simulink model "Michaels_CVModel_fast8"  (R2020a)
settings: Solver=ode23  StartTime=0.0  StopTime=30  RelTol=1e-2  EnableMultiTasking=on
model workspace (MAT data in the model file):
  Eao = 1.88
  Eesla = 0.58
  Eeslvf = 5.2
  Eesra = 0.63
  Eesrvf = 1.75
  Emaxspt = 48.75
  Epa = 0.15
  Epu = 0.04
  Esa = 0.37
  Esv = 0.013
  Evc = 0.03
  GpLV = 0
  GpRR = 11
  GpRV = 0
  GpRsa = 0
  GpV0 = 0
  GsLV = 0.007
  GsRR = 11
  GsRV = 0.022
  GsRsa = -0.05
  GsV0 = 31
  Ka = 4.4
  Lao = 0.0022
  Lav = 0.000354
  Lmt = 7.697e-05
  Lpa = 7.697e-05
  Lpv = 0.0001043
  Ltc = 8.009e-05
  P0la = 0.5
  P0lvf = 0.98
  P0pcd = 0.5
  P0ra = 0.5
  P0rvf = 0.91
  P0spt = 0.46
  PV : AO (value not decoded)
  PVao = [327.9; 100.9]
  Rao = 0.28
  Rav = 0.02
  Rla2pu = 0.5
  Rmt = 0.01
  Rpa = 0.12
  Rpa_Vals = 0.12
  Rpu = 0.006
  Rpv = 0.02
  Rra = 0.012
  Rsa = 0.74
  Rsv = 0.12
  Rtc = 0.01
  Tc = 1
  Tsys0 = 0.6
  V0la = 30
  V0lvf = 45
  V0pcd = 200
  V0ra = 25
  V0rvf = 50
  V0spt = 10
  Vdla = 15
  Vdlvf = 16
  Vdra = 15
  Vdrvf = 40
  Vdspt = 10
  Vlv0 = 100
  Vperi = 51
  Vrv0 = 105
  Vuao = 260.8
  Vupa = 91
  Vupu = 132
  Vusa = 287.4
  Vusv = 1976.1
  Vuvc = 136.17
  amin = -2
  artBrLVcontConti = []
  artBrLVcontDigi = [0 0 0 0 0 0 0 0 0 0 0 0 ... (240 elements, 1x240)]
  artBrRRConti = []
  artBrRRDigi = [0 0 0 0 0 0 0 0 0 0 1.57142857143 3.14285714286 ... (240 elements, 1x240)]
  artBrRVcontConti = []
  artBrRVcontDigi = [0 0 0 0 0 0 0 0 0 0 0 0 ... (240 elements, 1x240)]
  artBrRsaConti = []
  artBrRsaDigi = [0 0 0 0 0 0 0 0 0 0 0 0 ... (480 elements, 1x480)]
  artBrV0Conti = []
  artBrV0Digi = [0 0 0 0 0 0 0 0 0 0 0 0 ... (640 elements, 1x640)]
  atriumA = 1
  baroSampFreq = 16
  cP0la = 0.5
  cP0lvf = 0.98
  cP0ra = 0.5
  cP0rvf = 0.91
  cT = 1
  cVtotal = 5400
  clambdala = 0.13
  clambdalvf = 0.028
  clambdara = 0.13
  clambdarvf = 0.028
  deac = 0.0004
  ksys = 0.075
  lambdala = 0.065
  lambdalvf = 0.042
  lambdapcd = 0.005
  lambdara = 0.065
  lambdarvf = 0.028
  lambdaspt = 0.4
  pThor = 0
  params : object (value not decoded)
  sampleTime = 0.005
  svcPressureChange_MCS = 0
  svrMult = 1
  tStepOn = 1000000000
  t_baroOn = 1000000
  t_testBed_start = 1000000
  venk1 = 0.5
  venk2 = 0.5
symbols that are objects in the model workspace (value not decoded): PV
undefined symbols (not defined in the file): dfilt
libraries: simulink x85, fl_lib x39, nesl_utility x24, cstblocks x9, dspstat3 x9, dspobslib x5, SimscapeFluids_lib x5, sh_lib x1
(part 2 of 5)

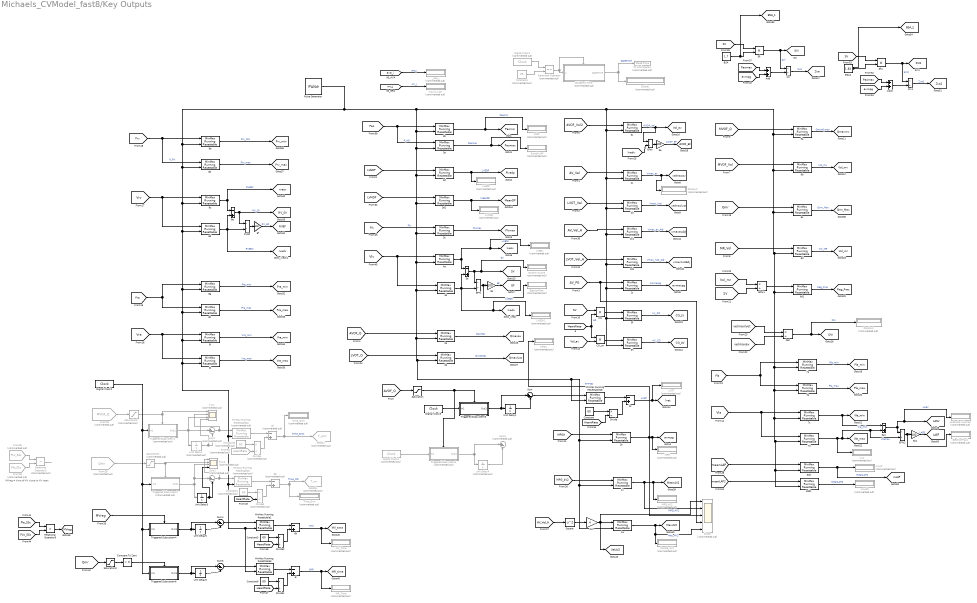
== system Michaels_CVModel_fast8/Key Outputs ==
  note: MRreg = time of MV close to MV open
  00 Date & Time : Subsystem  Commented=on
  1a : Sum  Description=1a  Inputs=-+
  1b : simulink/Math Operations/MinMax Running Resettable  Description=1b  Function=max  vinit=0
  1c : simulink/Math Operations/MinMax Running Resettable  Description=1c  Function=max  vinit=0
  1v : simulink/Math Operations/MinMax Running Resettable  Description=1b  Function=max  vinit=0
  1w : simulink/Math Operations/MinMax Running Resettable  Description=1b  Function=max  vinit=0
  1zv : Product  Inputs=*/
  1zv1 : Product  Inputs=*/
  2a : simulink/Math Operations/MinMax Running Resettable  Description=2a  Function=max  vinit=0
  2b : simulink/Math Operations/MinMax Running Resettable  Description=2b  Function=max  vinit=0
  2c : simulink/Math Operations/MinMax Running Resettable  Description=2c  Function=max  vinit=0
  2c1 : simulink/Math Operations/MinMax Running Resettable  Description=2c  Function=max  vinit=0
  2d : simulink/Math Operations/MinMax Running Resettable  Description=2d  Function=max  vinit=0
  2d1 : simulink/Math Operations/MinMax Running Resettable  Description=2d  Function=max  vinit=0
  2e0 : Product  Description=2e  Inputs=*/
  3a : simulink/Math Operations/MinMax Running Resettable  Description=3a  Function=max  vinit=0
  3b : simulink/Math Operations/MinMax Running Resettable  Description=3b  Function=min  vinit=250
  3c : simulink/Math Operations/MinMax Running Resettable  Description=3c  Function=max  vinit=0
  3d : simulink/Math Operations/MinMax Running Resettable  Description=3d  Function=max  vinit=0
  3d1 : simulink/Math Operations/MinMax Running Resettable  Description=3d  Function=max  vinit=0
  3dd : simulink/Math Operations/MinMax Running Resettable  Description=7d  Function=max  vinit=0
  3dd1 : simulink/Math Operations/MinMax Running Resettable  Description=7d  Function=max  vinit=0
  4V2 : Gain  Gain=4
  4a : simulink/Math Operations/MinMax Running Resettable  Description=4a  Function=min  vinit=250
  4b : simulink/Math Operations/MinMax Running Resettable  Description=4b  Function=max  vinit=0
  5a : Sum  Description=5a  Inputs=-+
  5a1 : Sum  Description=5a  Inputs=-+
  5b : Gain  Description=5b  Gain=100
  5b1 : Gain  Description=5b  Gain=100
  5c : simulink/Math Operations/MinMax Running Resettable  Description=5c  Function=max  vinit=0
  5e : Gain  Description=5e  Gain=100
  5f : simulink/Math Operations/MinMax Running Resettable  Description=5f  Function=max  vinit=0
  5fi : Product  Inputs=**
  5fi1 : Product  Inputs=**
  5h : simulink/Math Operations/MinMax Running Resettable  Description=5h  Function=max  vinit=0
  6a : simulink/Math Operations/MinMax Running Resettable  Description=6a  Function=max  vinit=0
  6b : simulink/Math Operations/MinMax Running Resettable  Description=6b  Function=max  vinit=0
  6c : simulink/Math Operations/MinMax Running Resettable  Description=6a  Function=max  vinit=0
  6d : simulink/Math Operations/MinMax Running Resettable  Description=6c  Function=max  vinit=0
  6d1 : simulink/Math Operations/MinMax Running Resettable  Description=6d  Function=max  vinit=0
  6f : Sum  Description=6f  Commented=on  Inputs=-+
  6g : Sum  Description=6g  Commented=on  Inputs=-+
  6h : Sum  Description=1a  Inputs=-+
  6i : Sum  Description=1a  Inputs=-+
  7a : simulink/Math Operations/MinMax Running Resettable  Description=7a  Function=min  vinit=250
  7b : simulink/Math Operations/MinMax Running Resettable  Description=7b  Function=max  vinit=0
  7c : simulink/Math Operations/MinMax Running Resettable  Description=7c  Function=min  vinit=250
  7d : simulink/Math Operations/MinMax Running Resettable  Description=7d  Function=max  vinit=0
  8a : simulink/Math Operations/MinMax Running Resettable  Description=3b  Function=min  vinit=250
  8b : simulink/Math Operations/MinMax Running Resettable  Description=3a  Function=max  vinit=0
  8c : simulink/Math Operations/MinMax Running Resettable  Description=4a  Function=min  vinit=250
  8d : simulink/Math Operations/MinMax Running Resettable  Description=4b  Function=max  vinit=0
  8e : Sum  Description=5a  Inputs=-+
  8f : Gain  Description=5b  Gain=100
  8g : simulink/Math Operations/MinMax Running Resettable  Description=7a  Function=min  vinit=250
  8h : simulink/Math Operations/MinMax Running Resettable  Description=7b  Function=max  vinit=0
  8i : simulink/Math Operations/MinMax Running Resettable  Description=7c  Function=min  vinit=250
  8j : simulink/Math Operations/MinMax Running Resettable  Description=7d  Function=max  vinit=0
  Add : Sum
  Add1 : Sum
  BSA : Constant  Value=1.7  SampleTime=0.001
  BSA2 : Constant  Value=1.83  SampleTime=0.001
  CO : Product  Inputs=**
  CO_av : Product  Inputs=**
  Compare To Zero : simulink/Logic and Bit Operations/Compare To Zero  relop=>  OutDataTypeStr=boolean  ZeroCross=off
  Constant : Constant  Value=60  SampleTime=0.001
  Constant1 : Constant  Commented=on  Value=60  SampleTime=0.001
  Constant3 : Constant  Value=60  SampleTime=0.001
  Constant4 : Constant  Commented=on  Value=25  SampleTime=0.001
  Constant5 : Constant  Commented=on  Value=60  SampleTime=0.001
  Constant6 : Constant  Value=60  SampleTime=0.001
  D BP : Display  Commented=on
  Digital Clock1 : DigitalClock  Commented=on  SampleTime=0.001
  Digital Clock2 : DigitalClock  SampleTime=0.001
  Digital Clock3 : DigitalClock  SampleTime=0.001
  Digital Clock4 : DigitalClock  Commented=on  SampleTime=0.001
  Display : Display  Commented=on
  Display1 : Display  Commented=on
  Display2 : Display  Commented=on
  Divide : Product  Inputs=*/
  Divide1 : Product  Inputs=*/
  Divide2 : Product  Inputs=*/
  Divide3 : Product  Commented=on  Inputs=*/
  Divide4 : Product  Commented=on  Inputs=*/
  EF% : Product  Inputs=*/
  EF%1 : Product  Inputs=*/
  EF%2 : Product  Inputs=*/
  EFav : Product  Inputs=*/
  EjectionFrac : Display  Commented=on
  EjectionFrac1 : Display  Commented=on
  From28 : From  Commented=on  GotoTag=Qmr  TagVisibility=global
  From29 : From  Commented=on  GotoTag=MVOF_Q  TagVisibility=global
  From35 : From  Commented=on  GotoTag=PLV_SSc  TagVisibility=global
  From36 : From  Commented=on  GotoTag=Pla_SSc  TagVisibility=global
      settings: CloseFcn=tagdialog Close
  From50 : From  Commented=on  GotoTag=HeartRate  TagVisibility=global
  Goto15 : Goto  Commented=on  GotoTag=T_mr  TagVisibility=global
  Goto17 : Goto  Commented=on  GotoTag=T_qmt  TagVisibility=global
  LAStroke Volume1 : Display  Commented=on
  LVEDP : Display  Commented=on
  LVEDV1 : Display  Commented=on
  LVESV : Display  Commented=on
  LVET : Display  Commented=on
  LVMDP : Display  Commented=on
  MPG : Display  Commented=on
  MPG1 : Display  Commented=on
  MPG_4V2 : Display  Commented=on
  MR_Time : Display  Commented=on
  MV_Time : Display  Commented=on
  MaxPG_4V2 : Display  Commented=on
  MinMax Running Resettable1 : simulink/Math Operations/MinMax Running Resettable  Function=max  vinit=0
  MinMax Running Resettable18 : simulink/Math Operations/MinMax Running Resettable  Function=max  vinit=0
  MinMax Running Resettable2 : simulink/Math Operations/MinMax Running Resettable  Commented=on  Function=max  vinit=0
  MinMax Running Resettable22 : simulink/Math Operations/MinMax Running Resettable  Commented=on  Function=max  vinit=0
  MinMax Running Resettable3 : simulink/Math Operations/MinMax Running Resettable  Function=max  vinit=0
  Pulse Generator : DiscretePulseGenerator  PulseType=Time based  Period=20  PhaseDelay=28.7
  RVEF : Product  Inputs=*/
  Relational Operator : RelationalOperator  Commented=on  Operator===  OutDataTypeStr=boolean  RndMeth=Simplest
  Relational Operator3 : RelationalOperator  Commented=on  Operator=>  OutDataTypeStr=boolean  RndMeth=Simplest
  Relational Operator5 : RelationalOperator  Operator=>  OutDataTypeStr=boolean  ZeroCross=off  RndMeth=Simplest
  Saturation : Saturate  UpperLimit=inf  LowerLimit=0  RndMeth=Ceiling
  Saturation1 : Saturate  Commented=on  UpperLimit=inf  LowerLimit=0  RndMeth=Ceiling
  Saturation2 : Saturate  UpperLimit=inf  LowerLimit=0  RndMeth=Ceiling
  Saturation3 : Saturate  Commented=on  UpperLimit=inf  LowerLimit=0  RndMeth=Ceiling
  Scope : Scope  Commented=on  NumInputPorts=5
  Square : Math  Operator=square  SaturateOnIntegerOverflow=on
  Stroke Volume : Display  Commented=on
  Sum : Sum  Inputs=|+-
  Sum1 : Sum  Commented=on  Inputs=|+-
  Sum2 : Sum  Commented=on  Inputs=|+-
  Sum3 : Sum  Commented=on  Inputs=|+-
  Sum4 : Sum  Inputs=|+-
  Sum5 : Sum  Inputs=|+-
  Systolic BP : Display  Commented=on
  T MV : Scope  Commented=on  NumInputPorts=4
  Time_Qmr : Display  Commented=on
  Time_Qmt : Display  Commented=on
  Tmr0 : Scope  Commented=on  NumInputPorts=4
  To Workspace1 : ToWorkspace  Commented=on  VariableName=DateTime  SaveFormat=Structure  SampleTime=1
      settings: MaxDataPoints=1  Save2DSignal=2-D array (concatenate along first dimension)
  Triggered Subsystem1 : Subsystem  Commented=on  TreatAsAtomicUnit=on
  Triggered Subsystem2 : Subsystem  Commented=on  TreatAsAtomicUnit=on
  Triggered Subsystem3 : Subsystem  Commented=on  TreatAsAtomicUnit=on
  Triggered Subsystem4 : Subsystem  TreatAsAtomicUnit=on
  Triggered Subsystem5 : Subsystem  TreatAsAtomicUnit=on
  Triggered Subsystem6 : Subsystem  TreatAsAtomicUnit=on
  Unit Delay{1,3,5..6} (4 alike) : UnitDelay  SampleTime=0.001
  Unit Delay2 : UnitDelay  Commented=on  SampleTime=0.001
  Unit Delay4 : UnitDelay  Commented=on  SampleTime=-1
  VLA : Display  Commented=on
  _ava_i : Display  Commented=on
  mLAP : Display  Commented=on
  mLAP2 : Display  Commented=on
  max(u,y)20 : Display  Commented=on
  tag scope: AVOF_EF=global, BSA_1=global, BSA_2=global, CO_AV=global, CO_LV=global, DVI=global, EF=global, LAEF=global, LASV=global, MR_time=global, MV_time=global, MVreg=global, Max4V2=global, Mean4V2=global, MeanDP=global, Paomax=global, Paomin=global, Pla_max=global, Pla_min=global, Plvedp=global, Plvmax=global, Pra_max=global, Pra_min=global, Prv_max=global, Prv_min=global, Qmaxav=global, Qmaxlvot=global, Qmaxmv=global, Qmr_Max=global, RVEF=global, RV_SV=global, Reg_Frac=global, SV=global, SVI2=global, SVI=global, Vel4V2=global, Vla_max=global, Vla_min=global, Vol_av=global, Vol_mr=global, Vol_mv=global, Vra_max=global, Vra_min=global, Zva2=global, Zva=global, avmaxpg=global, avmpg=global, lvedv=global, lvesv=global, lvet=global, mLAP=global, rvedv=global, rvesv=global, velmaxav=global, velmaxlvot=global, vmaxavAdj=global, vmaxlvotAdj=global
  wires:
  3c/1 -> [Plvmax]  "Plvmax"
  [Vlv] -> 4a/1, 4b/1
  4a/1 -> 5a/1, LVESV/1, [lvesv]  "LVESV"
  [LVOT_Vel] -> 2d/1
  [AV_Vel] -> 2c/1
  2a/1 -> [Qmaxav]  "QavMax"
  [AV_PG] -> Scope/4, 1c/1
  3a/1 -> Systolic BP/1, [Paomax]  "Paomax"
  2c/1 -> Display2/1, [velmaxav]  "Vmax_av"
  4b/1 -> 5a/2, LVEDV1/1, [lvedv], EF%/2  "LVEDV"
  [Plv] -> 3c/1  "Plv"
  3b/1 -> D BP/1, [Paomin]  "Paomin"
  [Pao] -> 3a/1, 3b/1  "P_AO"
  1c/1 -> [avmaxpg]  "AVmaxpg"
  6b/1 -> [Vol_mv]  "Vol_mv"
  6d/1 -> [Vol_mr]  "Vol_MR"
  5c/1 -> EFav/1, [Vol_av]  "AVOF_vol"
  [MVOF_Vol] -> 6b/1
  [AVOF_Vol2] -> 5c/1
  6a/1 -> [Qmaxmv]  "Qmvof_max"
  Triggered Subsystem5/1(Out1) -> Sum/1, Unit Delay1/1
  Unit Delay1/1 -> Sum/2
  [Pla] -> 7a/1, 7b/1
  7a/1 -> [Pla_min]  "Pla_min"
  7b/1 -> [Pla_max]  "Pla_max"
  [Vla] -> 7d/1, 7c/1
  Sum1/1 -> T MV/2, MinMax Running Resettable22/1
  Unit Delay2/1 -> T MV/4, Sum1/2
  [MVOF_Q] -> 6a/1
  Triggered Subsystem1/1(Out1) -> Unit Delay2/1, T MV/3, Sum1/1
  Triggered Subsystem2/1(Out1) -> Unit Delay3/1, Tmr0/3, Sum2/1
  [MR_Vol] -> 6d/1
  Unit Delay3/1 -> Tmr0/4, Sum2/2
  Sum2/1 -> MinMax Running Resettable2/1, Tmr0/1
  [AVOF_Q] -> Saturation/1
  MinMax Running Resettable18/1 -> 1a/1
  Sum/1 -> MinMax Running Resettable18/1
  [LVEDP] -> 3d/1
  3d/1 -> LVEDP/1, [Plvedp]  "LVEDP"
  Digital Clock4/1 -> Triggered Subsystem3/1(In1)
  Unit Delay4/1 -> Sum3/2
  Triggered Subsystem3/1(Out1) -> Sum3/1, Unit Delay4/1
  Constant/1 -> Divide/1
  1a/1 -> LVET/1, [lvet]  "LVET"
  [MPGX] -> 1b/1
  1b/1 -> MPG1/1, Scope/3, MPG/1, [avmpg]  "avmpg"
  2d/1 -> [velmaxlvot]  "Vmax_lvot"
  MinMax Running Resettable2/1 -> 6g/1
  Saturation1/1 -> Tmr0/2, Triggered Subsystem2/Trigger
  MinMax Running Resettable22/1 -> 6f/1
  Digital Clock3/1 -> Triggered Subsystem5/1(In1)
  5b/1 -> [EF]  "EF"
  EF%/1 -> EjectionFrac/1, 5b/1
  5a/1 -> EF%/1, [SV], Stroke Volume/1  "SV"
  [mr_j] -> max(u,y)20/1  "mr_j"
  [ava_i] -> _ava_i/1  "ava_i"
  6g/1 -> Goto15/1, Time_Qmr/1  "Time_MR"
  6f/1 -> Time_Qmt/1, Goto17/1  "Time_Qmt"
  7c/1 -> 5a1/1, [Vla_min]  "Vla_min"
  [AVOF_Q] -> 2a/1
  5f/1 -> [CO_LV]  "LV_CO"
  [SV] -> CO/1
  [Vol_av] -> CO_av/2
  5h/1 -> [CO_AV]  "AV_CO"
  [HeartRate] -> CO/2, CO_av/1  "HR"
  CO_av/1 -> 5h/1
  CO/1 -> 5f/1
  6d1/1 -> [Reg_Frac]  "Reg_Frac"
  EF%1/1 -> 6d1/1
  [Vol_mr] -> EF%1/1
  [SV] -> EF%1/2
  [velmaxlvot] -> 2e0/1
  [velmaxav] -> 2e0/2
  2e0/1 -> Display1/1, [DVI]  "DVI"
  [LVOT_Q] -> 2b/1
  2b/1 -> [Qmaxlvot]  "QlvotMax"
  5e/1 -> [AVOF_EF]  "AVOF_EF"
  EFav/1 -> 5e/1
  [lvedv] -> EFav/2
  8e/1 -> RVEF/1, [RV_SV]  "RV_SV"
  RVEF/1 -> 8f/1
  8d/1 -> 8e/2, [rvedv], RVEF/2  "RVEDV"
  8c/1 -> 8e/1, [rvesv]  "RVESV"
  8f/1 -> [RVEF]  "RV_EF"
  [Vrv] -> 8c/1, 8d/1
  8h/1 -> [Pra_max]  "Pra_max"
  [Pra] -> 8g/1, 8h/1
  8g/1 -> [Pra_min]  "Pra_min"
  [Vra] -> 8j/1, 8i/1
  8i/1 -> [Vra_min]  "Vra_min"
  8j/1 -> [Vra_max]  "Vra_max"
  [Prv] -> 8a/1, 8b/1  "P_RV"
  8a/1 -> [Prv_min]  "Prv_Min"
  8b/1 -> [Prv_max]  "Prv_max"
  From29/1 -> Saturation3/1
  From28/1 -> Saturation1/1
  [Qmr] -> 6c/1
  6c/1 -> [Qmr_Max]  "Qmr_Max"
  1v/1 -> Scope/2, [Mean4V2], MPG_4V2/1  "MPG_4V2"
  [MPG_4V2] -> 1v/1
  [AV_Vel_A] -> Square/1
  1w/1 -> Scope/5, MaxPG_4V2/1, [Max4V2]  "Max_4V2"
  4V2/1 -> [Vel4V2], Scope/1, 1w/1
  Square/1 -> 4V2/1
  2d1/1 -> [vmaxlvotAdj]  "Vmax_lvot_Adj"
  2c1/1 -> [vmaxavAdj]  "Vmax_av_Adj"
  [AV_Vel_A] -> 2c1/1
  [LVOT_Vel_A] -> 2d1/1
  3d1/1 -> [MeanDP], LVMDP/1  "meanDP"
  [LVMDP] -> 3d1/1
  Digital Clock1/1 -> Relational Operator/1
  Relational Operator/1 -> 00 Date & Time/Enable, 00 Date & Time/1(u)
  Constant4/1 -> Relational Operator/2
  00 Date & Time/1(DateTime) -> To Workspace1/1, Display/1  "DateTime"
  From35/1 -> Relational Operator3/1
  From36/1 -> Relational Operator3/2
  Relational Operator3/1 -> ?
  Saturation3/1 -> Triggered Subsystem1/Trigger, T MV/1
  6h/1 -> [MV_time], MV_Time/1  "tMV"
  [MVreg] -> Triggered Subsystem4/Enable
  Sum4/1 -> MinMax Running Resettable1/1
  MinMax Running Resettable1/1 -> 6h/1
  Unit Delay5/1 -> Sum4/2
  Triggered Subsystem4/1(Out1) -> Unit Delay5/1, Sum4/1
  [PLV_SSc] -> Relational Operator5/2
  [Pla_SSc] -> Relational Operator5/1
  Relational Operator5/1 -> [MVreg]
  Triggered Subsystem6/1(Out1) -> Sum5/1, Unit Delay6/1
  Unit Delay6/1 -> Sum5/2
  MinMax Running Resettable3/1 -> 6i/1
  Sum5/1 -> MinMax Running Resettable3/1
  Compare To Zero/1 -> Triggered Subsystem6/Enable
  6i/1 -> MR_Time/1, [MR_time]  "tMR"
  Digital Clock2/1 -> Triggered Subsystem6/1(In1), Triggered Subsystem4/1(In1), Triggered Subsystem2/1(In1), Triggered Subsystem1/1(In1)
  5fi/1 -> 1zv/1, [SVI]  "SVI"
  Add/1 -> 1zv/2
  BSA/1 -> [BSA_1], 5fi/2
  [SV] -> 5fi/1
  1zv/1 -> [Zva]  "Zva"
  [Paomax] -> Add/1
  [avmpg] -> Add/2
  [Qmr] -> Saturation2/1
  Saturation2/1 -> Compare To Zero/1
  Saturation/1 -> Triggered Subsystem5/Enable, Triggered Subsystem3/Trigger
  [HeartRate] -> Divide/2
  Divide/1 -> 1a/2
  5b1/1 -> [LAEF]  "LAEF"
  5a1/1 -> [LASV], LAStroke Volume1/1, EF%2/1  "LASV"
  7d/1 -> VLA/1, [Vla_max], EF%2/2, 5a1/2  "Vlamax"
  EF%2/1 -> EjectionFrac1/1, 5b1/1
  [meanLAP] -> 3dd/1
  3dd/1 -> [mLAP], mLAP/1  "meanLAP1"
  Divide1/1 -> 6i/2
  Constant6/1 -> Divide1/1
  [HeartRate] -> Divide1/2
  [HeartRate] -> Divide2/2
  Constant3/1 -> Divide2/1
  Divide2/1 -> 6h/2
  Divide3/1 -> 6g/2
  Constant1/1 -> Divide3/1
  [HeartRate] -> Divide3/2
  From50/1 -> Divide4/2
  Constant5/1 -> Divide4/1
  Divide4/1 -> 6f/2
  3dd1/1 -> mLAP2/1  "meanLAP2"
  [meanLAP2] -> 3dd1/1
  Pulse Generator/1 -> 3d1/2, 4a/2, 4b/2, 2a/2, MinMax Running Resettable18/2, 1v/2, 1w/2, 1b/2, 2b/2, 3c/2, 3d/2, 3a/2, 3b/2, 6c/2, 6d/2, 6d1/2, 7a/2, 7b/2, 3dd1/2, 3dd/2, 7d/2, 7c/2, 6b/2, 6a/2, 5c/2, 2d/2, 2c1/2, 2d1/2, 1c/2, 5h/2, 5f/2, 2c/2, 8g/2, 8h/2, MinMax Running Resettable22/2, MinMax Running Resettable1/2, MinMax Running Resettable3/2, MinMax Running Resettable2/2, 8j/2, 8i/2, 8d/2, 8c/2, 8b/2, 8a/2
  [avmpg] -> Add1/2
  [Paomax] -> Add1/1
  1zv1/1 -> [Zva2]  "Zva2"
  [SV] -> 5fi1/1
  Add1/1 -> 1zv1/2
  5fi1/1 -> [SVI2], 1zv1/1  "SVI2"
  BSA2/1 -> [BSA_2], 5fi1/2

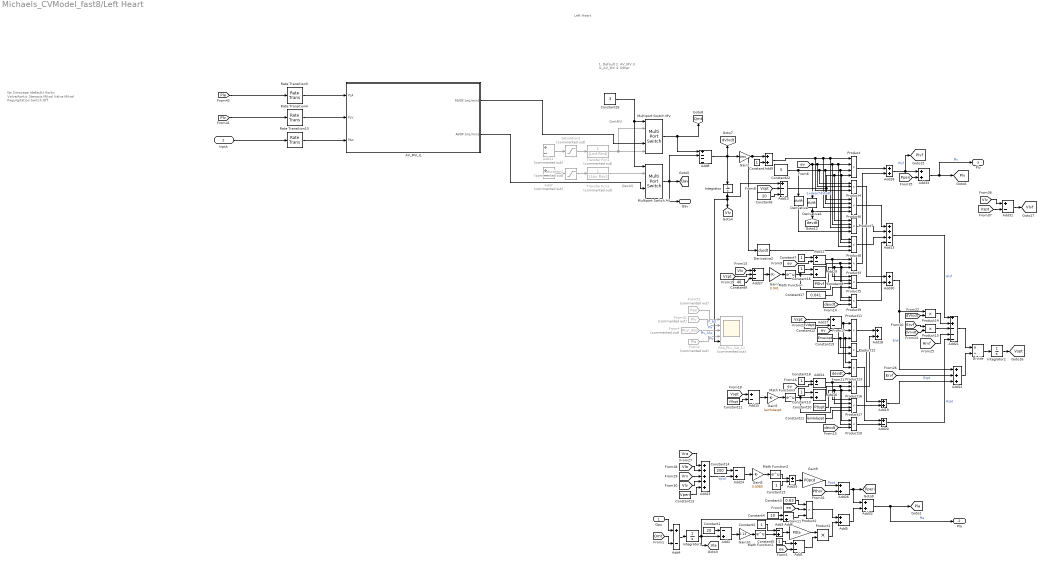
== system Michaels_CVModel_fast8/Left Heart ==
  note: No Simscape (default)
      | Aortic Valve/Aortic Stenosis
      | Mitral Valve
      | Mitral Regurgitation
      | Switch Off
  note: QavAS
  note: Left Heart
  note: QmtMV
  note: 1. Default
      | 2. AV_MV
      | 3. IL_AV_MV
      | 4. Other
  Qpu : Inport
  Input : Inport  Port=2
  AV_MV_IL : Subsystem
  Add{1,4,12,14..15,17,20,25,31} (9 alike) : Sum  Inputs=+-
  Add10 : Sum  Inputs=+--
  Add11 : Sum  Commented=on  Inputs=+-
  Add13 : Sum  Inputs=+++-
  Add{2..3,6,16,24,29} (6 alike) : Sum  Inputs=-+
  Add{5,9,18..19,26,28,30,32..33} (9 alike) : Sum
  Add21 : Sum  Inputs=++---
  Add22 : Sum  Inputs=+++
  Add23 : Sum  Inputs=+++++
  Add27 : Sum  Inputs=+--
  Add7 : Sum  Commented=on  Inputs=+-
  Add8 : Sum  Inputs=+---
  Constant{,2,5,7,10,15..16,18} (8 alike) : Constant
  Constant1 : Constant  Value=20
  Constant11 : Constant  Value=lambdaspt
  Constant12 : Constant  Value=Vdspt
  Constant13 : Constant  Value=Vperi
  Constant14 : Constant  Value=200
  Constant17 : Constant  Value=0.041
  Constant19 : Constant  Value=Emaxspt
  Constant20 : Constant  Value=P0spt
  Constant21 : Constant  Value=V0spt
  Constant22 : Constant  Value=5
  Constant26 : Constant  Value=3  SampleTime=-1
  Constant3 : Constant  Value=0.63
  Constant4 : Constant  Value=10
  Constant6 : Constant  Value=20
  Constant8 : Constant  Value=P0lvf
  Constant9 : Constant  Value=40
  Derivative : Derivative
  Derivative1 : Derivative
  Derivative2 : Derivative
  Divide : Product  Inputs=*/
  From2 : From  Commented=on  GotoTag=Pla  TagVisibility=global
      settings: CloseFcn=tagdialog Close
  From32 : From  Commented=on  GotoTag=Plv  TagVisibility=global
      settings: CloseFcn=tagdialog Close
  From4 : From  Commented=on  GotoTag=PLV_SSc  TagVisibility=global
      settings: CloseFcn=tagdialog Close
  From51 : From  Commented=on  GotoTag=Pao  TagVisibility=global
      settings: CloseFcn=tagdialog Close
  Gain10 : Gain  Gain=0.13
  Gain11 : Gain  Gain=P0la
  Gain2 : Gain  Gain=deac
  Gain3 : Gain  Gain=0.041
  Gain5 : Gain  Gain=lambdaspt
  Gain8 : Gain  Gain=0.0085
  Gain9 : Gain  Gain=P0pcd
  Integrator : Integrator  InitialCondition=140
  Integrator1 : Integrator  InitialCondition=40
  Integrator2 : Integrator  InitialCondition=20
  Math Function{,1..3} (4 alike) : Math  SignedPower=on  SaturateOnIntegerOverflow=on
  Multiport Switch AV : MultiPortSwitch  Inputs=4
  Multiport Switch MV : MultiPortSwitch  Inputs=4
  PAo_PLv_Vol_Lv : Scope  Commented=on  NumInputPorts=5
  Product{,5..8,17} (6 alike) : Product  Inputs=4  RndMeth=Zero
  Product{1,12,14..15} (4 alike) : Product  RndMeth=Zero
  Product{2..4,9..11,13,16} (8 alike) : Product  Inputs=3  RndMeth=Zero
  Rate Transition10 : RateTransition  OutPortSampleTimeMultiple=0.0  OutPortSampleTime=0.001
  Rate Transition3 : RateTransition  OutPortSampleTimeMultiple=0.0  OutPortSampleTime=0.001
  Rate Transition4 : RateTransition  OutPortSampleTimeMultiple=0.0  OutPortSampleTime=0.001
  Saturation1 : Saturate  Commented=on  UpperLimit=Inf  LowerLimit=0
  Saturation2 : Saturate  Commented=on  UpperLimit=Inf  LowerLimit=0
  Transfer Fcn1 : TransferFcn  Commented=on  Numerator=1  Denominator=[Lmt Rmt]
  Transfer Fcn2 : TransferFcn  Commented=on  Numerator=1  Denominator=[Lav Rav]
  Qav : Outport
  Pla : Outport  Port=2
  Plv : Outport  Port=3
  tag scope: Pla=global, Plv=global, Plvf=global, Pperi=global, Qav=global, Qmt=global, Vla=global, Vlv=global, Vlvf=global, Vspt=global, dVlvdt=global, devdt=global
  wires:
  Gain9/1 -> Add26/1  "Ppcd"
  [Pthor] -> Add26/2
  Add26/1 -> [Pperi], Add32/1
  Gain8/1 -> Math Function2/1
  Add24/1 -> Gain8/1
  Math Function2/1 -> Add25/1
  Constant15/1 -> Add25/2
  Add25/1 -> Gain9/1
  Math Function1/1 -> Add3/2
  Add3/1 -> Gain11/1
  Gain10/1 -> Math Function1/1
  Add2/1 -> Gain10/1
  Integrator1/1 -> Add2/2, Add6/2, [Vla]
  Constant1/1 -> Add2/1
  Add4/1 -> Integrator1/1
  Qpu/1 -> Add4/1
  [Qmt] -> Add4/2
  Constant2/1 -> Add3/1
  Constant4/1 -> Add6/1
  Add6/1 -> Product2/3
  [ea] -> Product2/2
  Constant3/1 -> Product2/1
  Product2/1 -> Add5/1
  Add5/1 -> Add32/2
  Add32/1 -> Pla/1, [Pla]  "Pla"
  Constant14/1 -> Add24/1
  [Vra] -> Add23/1
  [Vla] -> Add23/2
  [Vrv] -> Add23/3
  [Vlv] -> Add23/4
  Constant13/1 -> Add23/5
  Add23/1 -> Add24/2  "Vpcd"
  Gain11/1 -> Product1/1
  [ea] -> Add1/2
  Constant5/1 -> Add1/1
  Add1/1 -> Product1/2
  Product1/1 -> Add5/2
  Constant/1 -> Add9/2
  Gain2/1 -> Derivative2/1, Add9/1
  Add9/1 -> Product4/3, Product6/3, Product7/3, Product/1  "1+deac*dVlvdt"
  [ev] -> Product4/2, Product7/2, Product/2, Product8/3, Derivative1/1
  [Vspt] -> Add10/2
  Add10/1 -> Product7/1, Product/4, Product8/1, Product6/1
  Constant7/1 -> Add12/1
  Constant22/1 -> Product4/1, Product6/2, Product/3, Product8/2, Derivative/1
  [ev] -> Add12/2
  Product/1 -> Add28/1
  Product3/1 -> Add28/2
  Add28/1 -> Add33/1, [Plvf]  "Plvf"
  [Vlv] -> Add27/1
  [Vspt] -> Add27/2
  Constant9/1 -> Add27/3
  Gain3/1 -> Math Function/1
  Add27/1 -> Gain3/1
  Constant16/1 -> Add29/1
  Math Function/1 -> Add29/2, Product5/3
  Constant17/1 -> Product5/4
  Product4/1 -> Add30/1
  Product5/1 -> Add30/2
  Add30/1 -> Product14/1, Add22/1  "Elvf"
  Derivative1/1 -> Product6/4, [devdt]
  Derivative/1 -> Product7/4
  Constant8/1 -> Product5/2, Product3/3, Product9/1
  Add12/1 -> Product3/1, Product5/1
  Add29/1 -> Product3/2, Product9/2
  [devdt] -> Product9/3
  Product6/1 -> Add13/1
  Product7/1 -> Add13/2
  Product9/1 -> Add13/4
  Product8/1 -> Add13/3
  Add13/1 -> Add21/1  "Hlvf"
  Constant18/1 -> Add14/1
  [ev] -> Add14/2
  [Vspt] -> Add15/1
  Gain5/1 -> Math Function3/1
  Add15/1 -> Gain5/1
  Constant10/1 -> Add16/1
  Math Function3/1 -> Add16/2, Product17/3
  Constant11/1 -> Product17/4
  Constant20/1 -> Product17/2, Product16/3, Product10/1
  Add14/1 -> Product16/1, Product17/1
  Add16/1 -> Product16/2, Product10/2
  [devdt] -> Product10/3
  Constant21/1 -> Add15/2
  [ev] -> Product12/2, Product11/2
  Constant19/1 -> Product12/1, Product11/3, Product13/1
  [Vspt] -> Add17/1
  Constant12/1 -> Add17/2
  Add17/1 -> Product11/1, Product13/2
  [devdt] -> Product13/3
  Product11/1 -> Add18/1
  Product16/1 -> Add18/2
  Product12/1 -> Add19/1
  Product17/1 -> Add19/2
  Product13/1 -> Add20/1
  Product10/1 -> Add20/2
  Add19/1 -> Add22/3  "Espt"
  Add20/1 -> Add21/5  "Hspt"
  [dVlvdt] -> Product14/2
  Product15/1 -> Add21/3
  [Hrvf] -> Add21/4
  [Ervf] -> Add22/2
  Add21/1 -> Divide/1
  Add22/1 -> Divide/2
  Divide/1 -> Integrator2/1
  Integrator2/1 -> [Vspt]
  [Pperi] -> Add33/2
  Add33/1 -> Plv/1, [Plv]  "Plv"
  Saturation1/1 -> Transfer Fcn2/1
  Constant6/1 -> Add10/3
  Derivative2/1 -> Product8/4
  [Ervf] -> Product15/1
  [dVrvdt] -> Product15/2
  Product14/1 -> Add21/2
  Integrator/1 -> [Vlv], PAo_PLv_Vol_Lv/5, Add10/1
  Saturation2/1 -> Transfer Fcn1/1
  [Vlv] -> Add31/1
  [Vspt] -> Add31/2
  Add31/1 -> [Vlvf]
  Transfer Fcn2/1 -> Multiport Switch AV/2
  Transfer Fcn1/1 -> Multiport Switch MV/5, Multiport Switch MV/2
  Add7/1 -> Saturation1/1
  Add11/1 -> Saturation2/1
  Input/1 -> Rate Transition10/1
  [Pla] -> Rate Transition3/1
  [Plv] -> Rate Transition4/1
  From51/1 -> PAo_PLv_Vol_Lv/1  "P_AO"
  Constant26/1 -> Multiport Switch AV/1, Multiport Switch MV/1
  AV_MV_IL/1(MVOF [mL/min]) -> Multiport Switch MV/4
  AV_MV_IL/2(AVOF [mL/min]) -> Multiport Switch AV/4
  Multiport Switch AV/1 -> Add8/2, Qav/1, [Qav]
  Multiport Switch MV/1 -> [Qmt], Add8/1
  Rate Transition10/1 -> AV_MV_IL/3(PAo)
  Rate Transition4/1 -> AV_MV_IL/2(PLV)
  Rate Transition3/1 -> AV_MV_IL/1(PLA)
  From32/1 -> PAo_PLv_Vol_Lv/2  "Plv"
  From4/1 -> PAo_PLv_Vol_Lv/3  "Plv_SSc"
  From2/1 -> PAo_PLv_Vol_Lv/4  "Plv"
  Add8/1 -> Gain2/1, [dVlvdt], Integrator/1

== system Michaels_CVModel_fast8/Pulmonary ==
  note: Rla2pu = La to Pu reverse flow resistances resistance factor = 0.5.
      | NB: Pla to PPu Saturation set at 0.5.
  note: or Rpa = 0.06
  note: Pulmonary Circulation
  note: pv: pulmonary valve
      | pa: pulmonary peripheral vessels
      | pu, pulmonary veins
  Qpv : Inport
  Add{,4,6,8,20..21} (6 alike) : Sum  Inputs=+-
  Add1 : Sum  Inputs=-+
  Add2 : Sum
  Add3 : Sum
  Add5 : Sum  Inputs=-+
  Constant : Constant  Value=Vupa
  Constant2 : Constant  Value=Vupu
  Gain : Gain  Gain=0.15  SaturateOnIntegerOverflow=on
  Gain2 : Gain  Gain=0.04  SaturateOnIntegerOverflow=on
  Gain8 : Gain  Gain=Rla2pu  SaturateOnIntegerOverflow=on
  Integrator : Integrator  InitialCondition=12.9
  Integrator2 : Integrator  InitialCondition=280
  Pulmonary : Scope  Commented=on  NumInputPorts=7
  Rla2pu : Constant  Commented=on  Value=Rla2pu
  Saturation3 : Saturate  UpperLimit=Inf  LowerLimit=0.5
  Saturation4 : Saturate  UpperLimit=Inf  LowerLimit=0  ZeroCross=off
  Transfer Fcn7 : TransferFcn  Denominator=[Lpa Rpa]
  Transfer Fcn9 : TransferFcn  Denominator=[0.0000133 Rpu]
  Qpu : Outport
  Ppa : Outport  Port=2
  tag scope: Ppa=global, Ppu=global, Qpa=global, Qpu=global, Vpa=global, Vpu=global
  wires:
  Add/1 -> Integrator/1
  Integrator/1 -> Add1/2, [Vpa]
  Constant/1 -> Add1/1
  Add1/1 -> Gain/1
  Add4/1 -> Integrator2/1
  Add5/1 -> Gain2/1
  Qpv/1 -> Add/1
  Transfer Fcn7/1 -> Add/2, Add4/1, Pulmonary/2, [Qpa]  "Qpa"
  Constant2/1 -> Add5/1
  Integrator2/1 -> Add5/2, [Vpu]
  [Pthor2] -> Add2/1
  Add2/1 -> [Ppa], Pulmonary/5, Add6/1, Ppa/1  "Ppa"
  Gain/1 -> Add2/2
  [Pthor2] -> Add3/1
  Gain2/1 -> Add3/2  "Ppv"
  Add6/1 -> Transfer Fcn7/1
  Transfer Fcn9/1 -> Pulmonary/1, Add4/2, [Qpu], Qpu/1  "Qpu"
  Add3/1 -> Pulmonary/4, Add20/2, [Ppu], Add6/2, Add8/1  "PPu"
  [Pla] -> Pulmonary/3, Add20/1, Add8/2  "Pla"
  Add8/1 -> Pulmonary/7, Saturation4/1  "PPu - Pla"
  Gain8/1 -> Pulmonary/6, Add21/2  "Flow from LA to Pu"
  Saturation4/1 -> Add21/1
  Add20/1 -> Saturation3/1  "Pla-Ppu"
  Saturation3/1 -> Gain8/1
  Add21/1 -> Transfer Fcn9/1

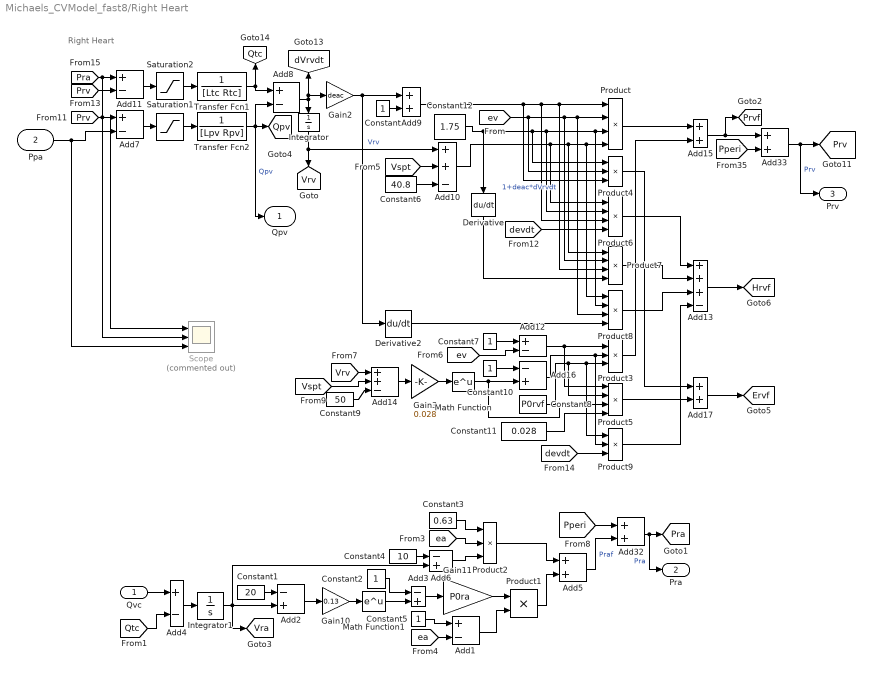
== system Michaels_CVModel_fast8/Right Heart ==
  note: Right Heart
  Qvc : Inport
  Ppa : Inport  Port=2
  Add{1,4,7..8,11..12} (6 alike) : Sum  Inputs=+-
  Add10 : Sum  Inputs=++-
  Add13 : Sum  Inputs=+++-
  Add14 : Sum  Inputs=++-
  Add{5,9,15,17,32..33} (6 alike) : Sum
  Add{2..3,6,16} (4 alike) : Sum  Inputs=-+
  Constant{,2,5,7,10} (5 alike) : Constant
  Constant1 : Constant  Value=20
  Constant11 : Constant  Value=0.028
  Constant12 : Constant  Value=1.75
  Constant3 : Constant  Value=0.63
  Constant4 : Constant  Value=10
  Constant6 : Constant  Value=40.8
  Constant8 : Constant  Value=P0rvf
  Constant9 : Constant  Value=50
  Derivative : Derivative
  Derivative2 : Derivative
  Gain10 : Gain  Gain=0.13
  Gain11 : Gain  Gain=P0ra
  Gain2 : Gain  Gain=deac
  Gain3 : Gain  Gain=0.028
  Integrator : Integrator  InitialCondition=100
  Integrator1 : Integrator  InitialCondition=60
  Math Function : Math  SignedPower=on  SaturateOnIntegerOverflow=on
  Math Function1 : Math  SignedPower=on  SaturateOnIntegerOverflow=on
  Product{,5..8} (5 alike) : Product  Inputs=4  RndMeth=Zero
  Product1 : Product  RndMeth=Zero
  Product{2..4,9} (4 alike) : Product  Inputs=3  RndMeth=Zero
  Saturation1 : Saturate  UpperLimit=Inf  LowerLimit=0
  Saturation2 : Saturate  UpperLimit=Inf  LowerLimit=0
  Scope : Scope  Commented=on  NumInputPorts=3
  Transfer Fcn1 : TransferFcn  Numerator=1  Denominator=[Ltc Rtc]
  Transfer Fcn2 : TransferFcn  Numerator=1  Denominator=[Lpv Rpv]
  Qpv : Outport
  Pra : Outport  Port=2
  Prv : Outport  Port=3
  tag scope: Ervf=global, Hrvf=global, Pra=global, Prv=global, Prvf=global, Qpv=global, Qtc=global, Vra=global, Vrv=global, dVrvdt=global
  wires:
  Math Function1/1 -> Add3/2
  Add3/1 -> Gain11/1
  Gain10/1 -> Math Function1/1
  Add2/1 -> Gain10/1
  Integrator1/1 -> Add2/2, Add6/2, [Vra]
  Constant1/1 -> Add2/1
  Add4/1 -> Integrator1/1
  Qvc/1 -> Add4/1
  [Qtc] -> Add4/2
  Constant2/1 -> Add3/1
  Constant4/1 -> Add6/1
  Add6/1 -> Product2/3
  [ea] -> Product2/2
  Constant3/1 -> Product2/1
  Product2/1 -> Add5/1
  Add5/1 -> Add32/2  "Praf"
  Add32/1 -> Pra/1, [Pra]  "Pra"
  Gain11/1 -> Product1/1
  [ea] -> Add1/2
  Constant5/1 -> Add1/1
  Add1/1 -> Product1/2
  Product1/1 -> Add5/2
  [Pperi] -> Add32/1
  Transfer Fcn1/1 -> Add8/1, [Qtc]
  Add8/1 -> Gain2/1, [dVrvdt], Integrator/1
  Constant/1 -> Add9/2
  Gain2/1 -> Add9/1, Derivative2/1
  Add9/1 -> Product4/3, Product6/3, Product7/3, Product/1  "1+deac*dVrvdt"
  [ev] -> Product4/2, Product7/2, Product/2, Product8/3
  [Vspt] -> Add10/2
  Add10/1 -> Product6/1, Product7/1, Product8/1, Product/4
  Constant7/1 -> Add12/1
  Constant12/1 -> Product4/1, Product6/2, Product/3, Product8/2, Derivative/1
  [ev] -> Add12/2
  Product/1 -> Add15/1
  Product3/1 -> Add15/2
  Add15/1 -> Add33/1, [Prvf]
  [Vrv] -> Add14/1
  [Vspt] -> Add14/2
  Constant9/1 -> Add14/3
  Gain3/1 -> Math Function/1
  Add14/1 -> Gain3/1
  Constant10/1 -> Add16/1
  Math Function/1 -> Add16/2, Product5/3
  Constant11/1 -> Product5/4
  Product4/1 -> Add17/1
  Product5/1 -> Add17/2
  Add17/1 -> [Ervf]
  Derivative/1 -> Product7/4
  Constant8/1 -> Product5/2, Product3/3, Product9/1
  Add12/1 -> Product3/1, Product5/1
  Add16/1 -> Product3/2, Product9/2
  Product6/1 -> Add13/1
  Product7/1 -> Add13/2
  Product9/1 -> Add13/4
  Product8/1 -> Add13/3
  Add13/1 -> [Hrvf]
  Add7/1 -> Saturation1/1
  Ppa/1 -> Scope/3, Add7/2
  [Pperi] -> Add33/2
  Add33/1 -> Prv/1, [Prv]  "Prv"
  Saturation1/1 -> Transfer Fcn2/1
  Constant6/1 -> Add10/3
  Derivative2/1 -> Product8/4
  Integrator/1 -> [Vrv], Add10/1  "Vrv"
  Add11/1 -> Saturation2/1
  [Prv] -> Add11/2
  [Pra] -> Scope/2, Add11/1
  Saturation2/1 -> Transfer Fcn1/1
  [devdt] -> Product6/4
  Transfer Fcn2/1 -> Qpv/1, Add8/2, [Qpv]  "Qpv"
  [devdt] -> Product9/3
  [Prv] -> Scope/1, Add7/1

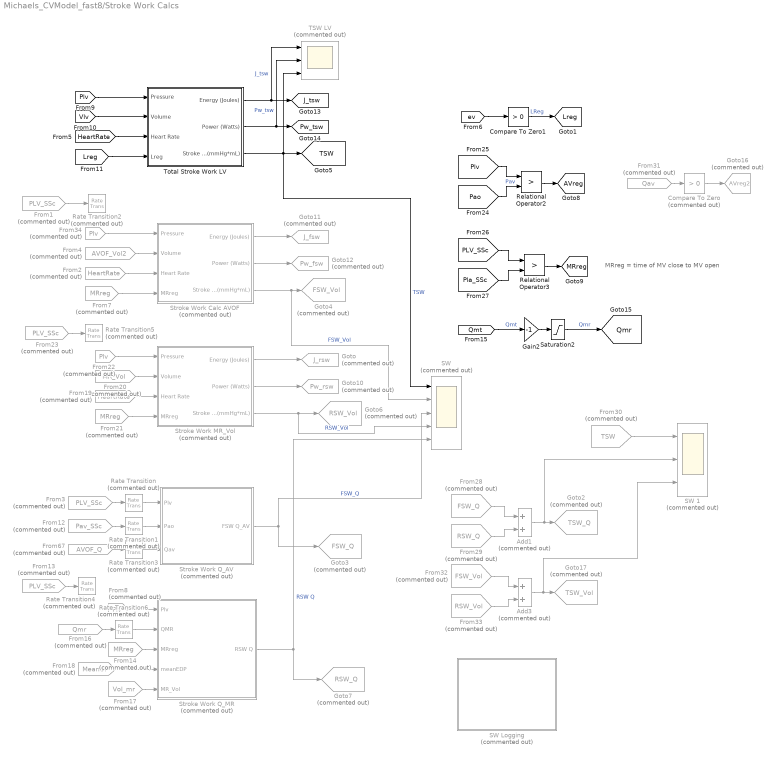
== system Michaels_CVModel_fast8/Stroke Work Calcs ==
  note: MRreg = time of MV close to MV open
  Add1 : Sum  Commented=on
  Add3 : Sum  Commented=on
  Compare To Zero : simulink/Logic and Bit Operations/Compare To Zero  Commented=on  relop=>  OutDataTypeStr=boolean
  Compare To Zero1 : simulink/Logic and Bit Operations/Compare To Zero  relop=>  OutDataTypeStr=boolean
  From{1,3,13,23} (4 alike) : From  Commented=on  GotoTag=PLV_SSc  TagVisibility=global
      settings: CloseFcn=tagdialog Close
  From12 : From  Commented=on  GotoTag=Pav_SSc  TagVisibility=global
      settings: CloseFcn=tagdialog Close
  From14 : From  Commented=on  GotoTag=MRreg  TagVisibility=global
      settings: CloseFcn=tagdialog Close
  From16 : From  Commented=on  GotoTag=Qmr  TagVisibility=global
      settings: CloseFcn=tagdialog Close
  From17 : From  Commented=on  GotoTag=Vol_mr  TagVisibility=global
      settings: CloseFcn=tagdialog Close
  From18 : From  Commented=on  GotoTag=MeanDP  TagVisibility=global
      settings: CloseFcn=tagdialog Close
  From19 : From  Commented=on  GotoTag=HeartRate  TagVisibility=global
      settings: CloseFcn=tagdialog Close
  From2 : From  Commented=on  GotoTag=HeartRate  TagVisibility=global
      settings: CloseFcn=tagdialog Close
  From20 : From  Commented=on  GotoTag=MR_Vol  TagVisibility=global
      settings: CloseFcn=tagdialog Close
  From21 : From  Commented=on  GotoTag=MRreg  TagVisibility=global
      settings: CloseFcn=tagdialog Close
  From22 : From  Commented=on  GotoTag=Plv  TagVisibility=global
      settings: CloseFcn=tagdialog Close
  From28 : From  Commented=on  GotoTag=FSW_Q  TagVisibility=global
  From29 : From  Commented=on  GotoTag=RSW_Q  TagVisibility=global
      settings: CloseFcn=tagdialog Close
  From30 : From  Commented=on  GotoTag=TSW  TagVisibility=global
  From31 : From  Commented=on  GotoTag=Qav  TagVisibility=global
      settings: CloseFcn=tagdialog Close
  From32 : From  Commented=on  GotoTag=FSW_Vol  TagVisibility=global
  From33 : From  Commented=on  GotoTag=RSW_Vol  TagVisibility=global
      settings: CloseFcn=tagdialog Close
  From34 : From  Commented=on  GotoTag=Plv  TagVisibility=global
      settings: CloseFcn=tagdialog Close
  From4 : From  Commented=on  GotoTag=AVOF_Vol2  TagVisibility=global
      settings: CloseFcn=tagdialog Close
  From67 : From  Commented=on  GotoTag=AVOF_Q  TagVisibility=global
      settings: CloseFcn=tagdialog Close
  From7 : From  Commented=on  GotoTag=MRreg  TagVisibility=global
      settings: CloseFcn=tagdialog Close
  From8 : From  Commented=on  GotoTag=Plv  TagVisibility=global
      settings: CloseFcn=tagdialog Close
  Gain2 : Gain  Gain=-1
  Goto : Goto  Commented=on  GotoTag=J_rsw  TagVisibility=global
  Goto10 : Goto  Commented=on  GotoTag=Pw_rsw  TagVisibility=global
  Goto11 : Goto  Commented=on  GotoTag=J_fsw  TagVisibility=global
  Goto12 : Goto  Commented=on  GotoTag=Pw_fsw  TagVisibility=global
  Goto16 : Goto  Commented=on  GotoTag=AVreg2  TagVisibility=global
  Goto17 : Goto  Commented=on  GotoTag=TSW_Vol  TagVisibility=global
  Goto2 : Goto  Commented=on  GotoTag=TSW_Q  TagVisibility=global
  Goto3 : Goto  Commented=on  GotoTag=FSW_Q  TagVisibility=global
  Goto4 : Goto  Commented=on  GotoTag=FSW_Vol  TagVisibility=global
  Goto6 : Goto  Commented=on  GotoTag=RSW_Vol  TagVisibility=global
  Goto7 : Goto  Commented=on  GotoTag=RSW_Q  TagVisibility=global
  Rate Transition{,1..6} (7 alike) : RateTransition  Commented=on
  Relational Operator2 : RelationalOperator  Operator=>  OutDataTypeStr=boolean  ZeroCross=off  RndMeth=Simplest
  Relational Operator3 : RelationalOperator  Operator=>  OutDataTypeStr=boolean  RndMeth=Simplest
  "SW " : Scope  Commented=on  NumInputPorts=5
  SW 1 : Scope  Commented=on  NumInputPorts=3
  SW Logging : Subsystem  Description=Stroke Work  Commented=on
  Saturation2 : Saturate  UpperLimit=inf  LowerLimit=0
  Stroke Work Calc AVOF : Subsystem  Commented=on
  Stroke Work MR_Vol : Subsystem  Commented=on
  Stroke Work Q_AV : Subsystem  Commented=on
  Stroke Work Q_MR : Subsystem  Commented=on
  TSW LV : Scope  Commented=on  NumInputPorts=3
  Total Stroke Work LV : Subsystem
  tag scope: AVreg=global, J_tsw=global, Lreg=global, MRreg=global, Pw_tsw=global, Qmr=global, TSW=global
  wires:
  Rate Transition3/1 -> Stroke Work Q_AV/3(Qav)
  Rate Transition1/1 -> Stroke Work Q_AV/2(Pao)
  Stroke Work Q_AV/1(FSW Q_AV) -> Goto3/1, "SW "/3  "FSW_Q"
  From67/1 -> Rate Transition3/1
  From12/1 -> Rate Transition1/1
  From3/1 -> Rate Transition/1
  From7/1 -> Stroke Work Calc AVOF/4(MRreg)
  From2/1 -> Stroke Work Calc AVOF/3(Heart Rate)
  From4/1 -> Stroke Work Calc AVOF/2(Volume)
  From1/1 -> Rate Transition2/1
  Stroke Work Calc AVOF/3(Stroke Work (mmHg*mL)) -> "SW "/2, Goto4/1  "FSW_Vol"
  Total Stroke Work LV/3(Stroke Work (mmHg*mL)) -> "SW "/1, [TSW], TSW LV/3  "TSW"
  Total Stroke Work LV/2(Power (Watts)) -> [Pw_tsw], TSW LV/2  "Pw_tsw"
  [Vlv] -> Total Stroke Work LV/2(Volume)
  [HeartRate] -> Total Stroke Work LV/3(Heart Rate)
  Total Stroke Work LV/1(Energy (Joules)) -> [J_tsw], TSW LV/1  "J_tsw"
  [Lreg] -> Total Stroke Work LV/4(Lreg)
  [ev] -> Compare To Zero1/1
  Compare To Zero1/1 -> [Lreg]  "LReg"
  [Pla_SSc] -> Relational Operator3/2
  [PLV_SSc] -> Relational Operator3/1
  [Plv] -> Relational Operator2/1
  [Pao] -> Relational Operator2/2  "Pav"
  Relational Operator3/1 -> [MRreg]
  Relational Operator2/1 -> [AVreg]
  From13/1 -> Rate Transition4/1
  From16/1 -> Rate Transition6/1
  Rate Transition6/1 -> Stroke Work Q_MR/2(QMR)
  From14/1 -> Stroke Work Q_MR/3(MRreg)
  [Qmt] -> Gain2/1  "Qmt"
  Gain2/1 -> Saturation2/1
  Saturation2/1 -> [Qmr]  "Qmr"
  From17/1 -> Stroke Work Q_MR/5(MR_Vol)
  From19/1 -> Stroke Work MR_Vol/3(Heart Rate)
  From22/1 -> Stroke Work MR_Vol/1(Pressure)
  From21/1 -> Stroke Work MR_Vol/4(MRreg)
  From20/1 -> Stroke Work MR_Vol/2(Volume)
  From23/1 -> Rate Transition5/1
  Stroke Work MR_Vol/3(Stroke Work (mmHg*mL)) -> Goto6/1, "SW "/4  "RSW_Vol"
  Stroke Work Q_MR/1(RSW Q) -> Goto7/1, "SW "/5  "RSW Q"
  Stroke Work MR_Vol/2(Power (Watts)) -> Goto10/1
  Stroke Work MR_Vol/1(Energy (Joules)) -> Goto/1
  Stroke Work Calc AVOF/1(Energy (Joules)) -> Goto11/1
  Stroke Work Calc AVOF/2(Power (Watts)) -> Goto12/1
  From28/1 -> Add1/1
  From29/1 -> Add1/2
  Add1/1 -> SW 1/2, Goto2/1
  From33/1 -> Add3/2
  From32/1 -> Add3/1
  Add3/1 -> SW 1/3, Goto17/1
  Compare To Zero/1 -> Goto16/1
  From31/1 -> Compare To Zero/1
  Rate Transition/1 -> Stroke Work Q_AV/1(Plv)
  From8/1 -> Stroke Work Q_MR/1(Plv)
  From30/1 -> SW 1/1
  [Plv] -> Total Stroke Work LV/1(Pressure)
  From18/1 -> Stroke Work Q_MR/4(meanEDP)
  From34/1 -> Stroke Work Calc AVOF/1(Pressure)

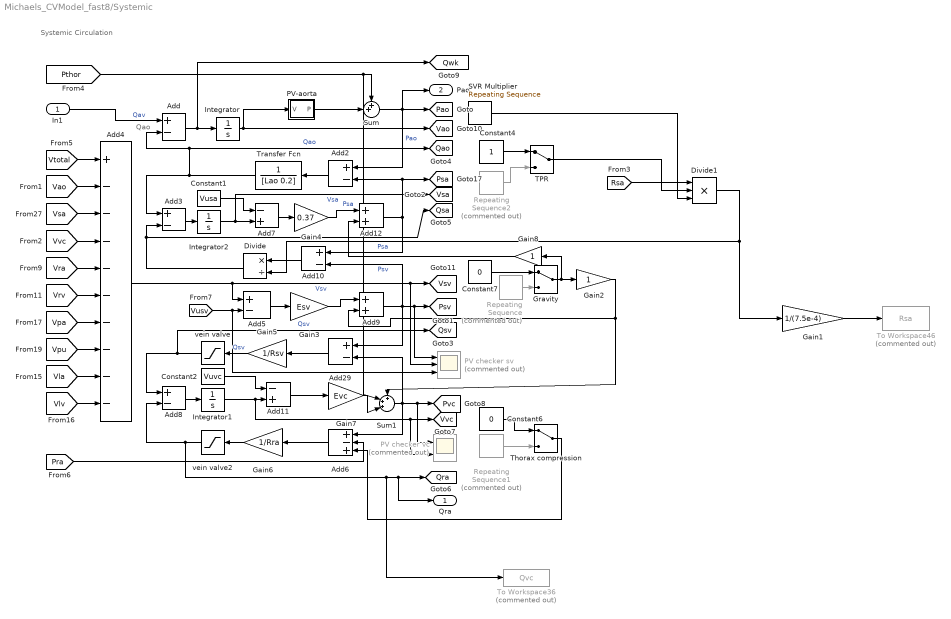
== system Michaels_CVModel_fast8/Systemic ==
  note: Systemic Circulation
  note: Qao
  In1 : Inport
  Add{,2..3,5,8,10,29} (7 alike) : Sum  Inputs=+-
  Add11 : Sum  Inputs=-+
  Add12 : Sum
  Add4 : Sum  Inputs=+---------
  Add6 : Sum  Inputs=+-+
  Add7 : Sum  Inputs=-+
  Add9 : Sum
  Constant1 : Constant  Value=Vusa
  Constant2 : Constant  Value=Vuvc
  Constant4 : Constant
  Constant6 : Constant  Value=0
  Constant7 : Constant  Value=0
  Divide : Product  Inputs=*/
  Divide1 : Product  Inputs=***
  Gain1 : Gain  Gain=1/(7.5e-4)
  Gain2 : Gain
  Gain3 : Gain  Gain=Esv
  Gain4 : Gain  Gain=0.37
  Gain5 : Gain  Gain=1/Rsv
  Gain6 : Gain  Gain=1/Rra
  Gain7 : Gain  Gain=Evc
  Gain8 : Gain
  Gravity : ManualSwitch
  Integrator : Integrator  InitialCondition=180
  Integrator1 : Integrator  InitialCondition=760
  Integrator2 : Integrator  InitialCondition=760
  PV checker sv : Scope  Commented=on  NumInputPorts=3
  PV checker vc : Scope  Commented=on  NumInputPorts=2
  PV-aorta : Subsystem
  Repeating Sequence : simulink/Sources/Repeating Sequence  Commented=on  rep_seq_t=[0 7 13 200]  rep_seq_y=[0 0 -10 -10]
  Repeating Sequence1 : simulink/Sources/Repeating Sequence  Commented=on  rep_seq_t=[0 10 11 20 21 200]  rep_seq_y=[0 0 10 10 0 0]
  Repeating Sequence2 : simulink/Sources/Repeating Sequence  Commented=on  rep_seq_t=[0 10 11 15 22 200]  rep_seq_y=[1 1 0.4 0.4 1 1]
  SVR Multiplier : simulink/Sources/Repeating Sequence  rep_seq_t=[0 59.5 60 119.5 120]  rep_seq_y=[1 1 svrMult svrMult 1]
  Sum : Sum  Inputs=++|
  Sum1 : Sum  Inputs=+++|
  TPR : ManualSwitch
  Thorax compression : ManualSwitch
  To Workspace36 : ToWorkspace  Commented=on  VariableName=Qvc  SampleTime=0.005
  To Workspace46 : ToWorkspace  Commented=on  VariableName=Rsa  SampleTime=0.005
  Transfer Fcn : TransferFcn  Denominator=[Lao 0.2]
  vein valve : Saturate  UpperLimit=inf  LowerLimit=0
  vein valve2 : Saturate  UpperLimit=inf  LowerLimit=0
  Qra : Outport
  Pao : Outport  Port=2
  tag scope: Pao=global, Psa=global, Psv=global, Pvc=global, Qao=global, Qra=global, Qsa=global, Qsv=global, Qwk=global, Vao=global, Vsa=global, Vsv=global, Vvc=global
  wires:
  In1/1 -> Add/1  "Qav"
  Add/1 -> [Qwk], Integrator/1
  Integrator/1 -> PV-aorta/1(V), [Vao]
  Add7/1 -> Gain4/1
  Add12/1 -> Add10/1, Add2/2, [Psa]  "Psa"
  Transfer Fcn/1 -> Add3/1, Add/2, [Qao]  "Qao"
  Add29/1 -> Gain5/1
  [Vao] -> Add4/2
  Add5/1 -> Gain3/1
  [Vsa] -> Add4/3
  [Vtotal] -> Add4/1
  [Vvc] -> Add4/4
  [Vra] -> Add4/5
  [Vrv] -> Add4/6
  [Vusv] -> Add5/2, PV checker sv/3
  [Pra] -> Add6/2
  Gain5/1 -> vein valve/1  "Qsv"
  Integrator2/1 -> Add7/2, [Vsa]  "Vsa"
  Constant1/1 -> Add7/1
  Add3/1 -> Integrator2/1
  Add8/1 -> Integrator1/1
  Add11/1 -> Gain7/1
  Constant2/1 -> Add11/1
  Integrator1/1 -> Add11/2, [Vvc], PV checker vc/2
  Add6/1 -> Gain6/1
  Gain6/1 -> vein valve2/1
  Add2/1 -> Transfer Fcn/1
  Add10/1 -> Divide/1
  Divide/1 -> Add3/2, [Qsa]
  Add4/1 -> Add5/1, [Vsv], PV checker sv/2  "Vsv"
  [Vpa] -> Add4/7
  [Vpu] -> Add4/8
  [Vla] -> Add4/9
  [Vlv] -> Add4/10
  vein valve/1 -> Add8/1, [Qsv]  "Qsv"
  vein valve2/1 -> Add8/2, To Workspace36/1, Qra/1, [Qra]
  [Pthor] -> Sum/1, Sum1/2
  PV-aorta/1(P) -> Sum/2
  Sum/1 -> [Pao], Add2/1, Pao/1  "Pao"
  Sum1/1 -> Add6/1, Add29/2, [Pvc], PV checker vc/1
  Add9/1 -> Add29/1, Add10/2, [Psv], PV checker sv/1  "Psv"
  Gain7/1 -> Sum1/3
  Divide1/1 -> Gain1/1, Divide/2
  Gain1/1 -> To Workspace46/1
  Constant4/1 -> TPR/1
  Repeating Sequence2/1 -> TPR/2
  TPR/1 -> Divide1/2
  Constant7/1 -> Gravity/1
  Repeating Sequence/1 -> Gravity/2
  Constant6/1 -> Thorax compression/1
  Repeating Sequence1/1 -> Thorax compression/2
  Gain4/1 -> Add12/1  "Psa"
  Gravity/1 -> Gain8/1, Gain2/1
  Gain2/1 -> Add9/2, Sum1/1
  Gain8/1 -> Add12/2
  Thorax compression/1 -> Add6/3
  SVR Multiplier/1 -> Divide1/3
  Gain3/1 -> Add9/1
  [Rsa] -> Divide1/1

== system Michaels_CVModel_fast8/Thoracic Pressure And Breathing ==
  note: Closed or open chest
  note: Breathing
  note: 1. Off
      | 2. On
  Breathing sinusoidal : Subsystem  Commented=on
  Compare To Constant : simulink/Logic and Bit Operations/Compare To Constant  relop===  const=3.0  OutDataTypeStr=uint8
  Constant3 : Constant  Value=0
  Multiport Switch : MultiPortSwitch
  Product : Product  RndMeth=Zero
  Pthor : Constant  Value=0
  Pthor2Select : Constant
  valsalva : simulink/Sources/Repeating Sequence  Commented=on  rep_seq_t=[0 59.5 60 89.5 90]  rep_seq_y=[0 0 pThor pThor 0]
  tag scope: Pthor2=global, Pthor=global, pValsalva=global
  wires:
  Multiport Switch/1 -> [Pthor2]
  Constant3/1 -> Multiport Switch/2
  Pthor2Select/1 -> Multiport Switch/1, Compare To Constant/1
  Breathing sinusoidal/1(Out1) -> Multiport Switch/3
  Pthor/1 -> [Pthor]  "PthorpT"
  valsalva/1 -> Multiport Switch/4, Product/2
  Compare To Constant/1 -> Product/1
  Product/1 -> [pValsalva]

== system Michaels_CVModel_fast8/Variables to Workspace ==
  CVtotal : Sum  Inputs=+-
  Constant2 : Constant  Value=5200
  Constant9 : Constant  Value=0
  Flow : Subsystem  Commented=on
  From39 : From  Commented=on  GotoTag=ev  TagVisibility=global
      settings: CloseFcn=tagdialog Close
  From40 : From  Commented=on  GotoTag=ea  TagVisibility=global
      settings: CloseFcn=tagdialog Close
  Key_Outputs_Link : Subsystem
  Pressure : Subsystem  Commented=on
  Settings : Subsystem  Description=Parameters  Commented=on
  To Workspace22 : ToWorkspace  VariableName=Vtotal  SampleTime=0.005
  To Workspace29 : ToWorkspace  Commented=on  VariableName=ev  SampleTime=0.005
  To Workspace30 : ToWorkspace  Commented=on  VariableName=ea  SampleTime=0.005
  To Workspace45 : ToWorkspace  VariableName=tt  SampleTime=0.005
  Volume : Subsystem
  tag scope: Vtotal=global
  wires:
  From39/1 -> To Workspace29/1
  From40/1 -> To Workspace30/1
  [Vtotal] -> To Workspace22/1
  CVtotal/1 -> [Vtotal]  "cvTotal"
  Constant2/1 -> CVtotal/1
  Constant9/1 -> CVtotal/2
  [tt] -> To Workspace45/1
